simulink model "ukol10"  (R2017b)
settings: Solver=VariableStepAuto  StartTime=0.0  StopTime=10.0  RelTol=1e-3
settings Model: Creator=ladislav  LastModifiedBy=ladislav

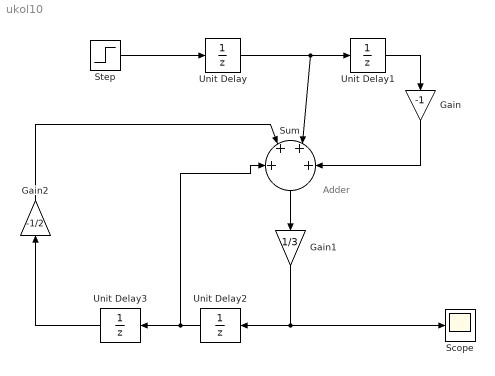
== system ukol10 ==
  note: Adder
  Gain : Gain  Gain=-1
  Gain1 : Gain  Gain=1/3
  Gain2 : Gain  Gain=-1/2
  "Scope " : Scope
  "Step " : Step  SampleTime=0
  Sum : Sum  Inputs=4
  "Unit Delay " : UnitDelay  SampleTime=-1
  "Unit Delay1 " : UnitDelay  SampleTime=-1
  "Unit Delay2 " : UnitDelay  SampleTime=-1
  "Unit Delay3 " : UnitDelay  SampleTime=-1
  wires:
  "Step "/1 -> "Unit Delay "/1
  "Unit Delay "/1 -> "Unit Delay1 "/1, Sum/3
  "Unit Delay1 "/1 -> Gain/1
  Sum/1 -> Gain1/1
  Gain1/1 -> "Scope "/1, "Unit Delay2 "/1
  Gain/1 -> Sum/4
  "Unit Delay3 "/1 -> Gain2/1
  "Unit Delay2 "/1 -> "Unit Delay3 "/1, Sum/1
  Gain2/1 -> Sum/2
